simulink model "Main_Sim_Kylle"  (R2018b)
settings: Solver=ode5  StartTime=0.0  StopTime=20000  FixedStep=simParams.sample_time_s  RelTol=1e-3  EnableMultiTasking=on
undefined symbols (not defined in the file or in its folder): DiscIntNeverNeededParam, FSW_Lib, fswParams, MEKF_lib, q_body, r_eci_km, satelliteDynamics_lib, simParams, v_eci_km, w_body_radps
libraries: vrlib x6, aerolibutil x5, CrossProdMatrix_lib x4, sharedutil x4, dspmathops x2, actuators_lib x1, CDH_command_lib x1, Environment_lib x1, MEKF_Conversion_lib x1, sharedtransform x1, actuator_processing_lib x1, allocation_lib x1
(part 2 of 2)

== matlab function Main_Sim_Kylle/FSW_Lib/MEKF_lib/Time Propagation of q & P_chol/If Action Subsystem/Time Propagation of P_chol via QR Decomposition ==
  data: P_sq input; Phi_discrete input; P_sq output; Q_sq input
function P_sq  = Cqr(P_sq,Phi_discrete,Q_sq)
%#codegen

A_QR2 = [P_sq'*Phi_discrete';Q_sq'];
         [~,R2] = qr(A_QR2);
          sq_P_kp1 = R2(1:6,1:6)';
          P_sq = sq_P_kp1;
end

== matlab function Main_Sim_Kylle/FSW_Lib/MEKF_lib/Measurement Update/QR Factorization ==
  data: P_sq output; R_sq input; K output; P_sq input; gyro_valid input; H input
function [P_sq,K] = A_QR(R_sq,P_sq, gyro_valid,H)
%#codegen
[nr,~] = size(R_sq);
[np,~] = size(P_sq);
A_QR = [R_sq',zeros(nr,np);(P_sq')*H', P_sq'];

[~,R] = qr(A_QR);
        P_sq = R(7:12,7:12)'; %Updated P_sq
        K_bar = R(1:6,7:12)';    
        Innovation_sq = R(1:6,1:6)';
        
        K = K_bar/(Innovation_sq);
        
        if( gyro_valid == 0 )
    K(4:6,:) = zeros(3,6); %this is done so that we do not update bias based
                            % on false gyro readings
        end
end

== matlab function Main_Sim_Kylle/FSW_Lib/MEKF_lib/Time Propagation of q & P_chol/Create State Transition Matrix ==
  data: om_mag input; omega_x input; dt input; Phi output
function Phi = Phi_disc(om_mag,omega_x,dt)
%#codegen
% State Transition Matrix
w_n     = om_mag;
w_skew  = omega_x;

if( w_n < 1e-10 )
    Phi = [ eye(3)     -eye(3)*dt;
            zeros(3,3)  eye(3) ];
else
    Phi_11  = eye(3) - w_skew*(sin(w_n*dt)/w_n) + ...
                                        w_skew^2*(1 - cos(w_n*dt))/w_n^2;
    Phi_12  = w_skew*(1 - cos(w_n*dt))/w_n^2 - eye(3)*dt - ...
                                    w_skew^2*(w_n*dt - sin(w_n*dt))/w_n^3;
    Phi_21  = zeros(3,3);    
    Phi_22  = eye(3);    
    Phi     = [ Phi_11 Phi_12;
                Phi_21 Phi_22 ];
end
